simulink model "Practica1_InmanArturoArmasSalas"  (R2024a)
settings: Solver=ode23  StartTime=0.0  StopTime=10  RelTol=1e-3
values from neighbouring files (symbols this model uses):
  g = 9.81    [ParametrosPendulo.m]    (also in condiciones.m)
  l1 = 0.3    [ParametrosPendulo.m]    (also in condiciones.m)
  l2 = 0.25    [ParametrosPendulo.m]    (also in condiciones.m)
  m1 = 0.2    [ParametrosPendulo.m]    (also in condiciones.m)
  m2 = 0.1    [ParametrosPendulo.m]    (also in condiciones.m)
settings Model: Creator=Charles  LastModifiedBy=Elasticsole57
settings SolverCC: AlgebraicLoopSolver=TrustRegion
settings DataIOCC: ReturnWorkspaceOutputs=off
settings DebuggingCC: UnconnectedInputMsg=warning  UnconnectedOutputMsg=warning  UnconnectedLineMsg=warning  ArithmeticOperatorsInVariantConditions=warning
settings ModelReferenceCC: EnableRefExpFcnMdlSchedulingChecks=on
settings SFSimCC: SimUseLocalCustomCode=off  CustomCodeUndefinedFunction=UseInterfaceOnly
settings RTWCC: RTWUseLocalCustomCode=off  GPUComputeCapability=3.5

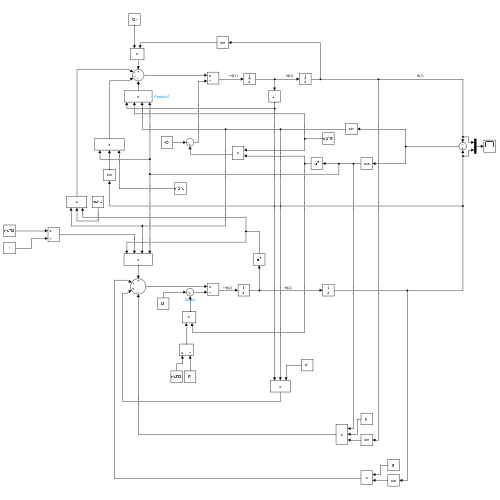
[thumbnail: Simulink's stored preview of the top-level diagram]
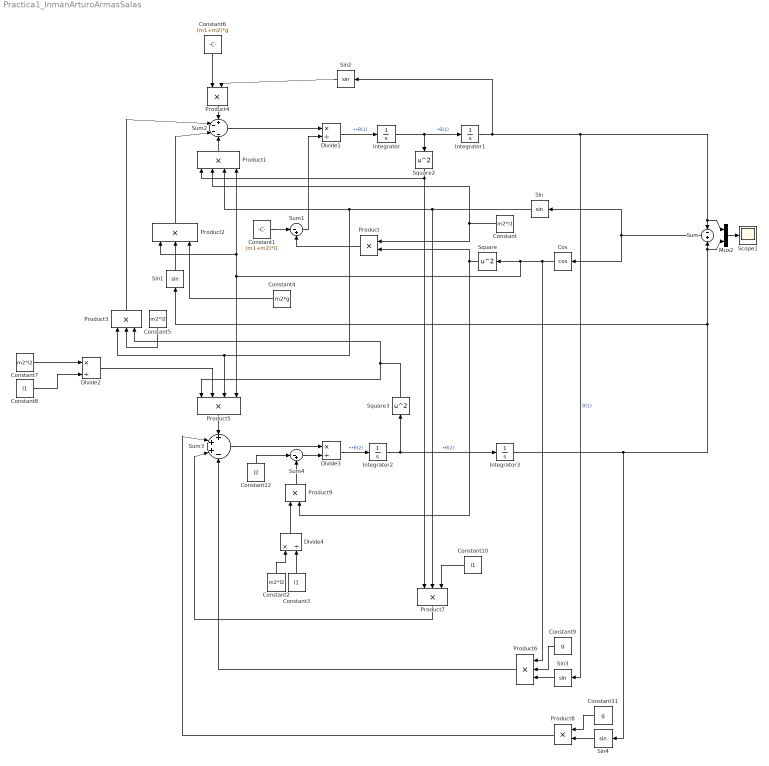
== system Practica1_InmanArturoArmasSalas ==
  Constant : Constant  Value=m2*l1
  Constant1 : Constant  Value=(m1+m2)*l1
  Constant10 : Constant  Value=l1
  Constant11 : Constant  Value=g
  Constant12 : Constant  Value=l2
  Constant2 : Constant  Value=m2*l2
  Constant3 : Constant  Value=l1
  Constant4 : Constant  Value=m2*g
  Constant5 : Constant  Value=m2*l2
  Constant6 : Constant  Value=(m1+m2)*g
  Constant7 : Constant  Value=m2*l2
  Constant8 : Constant  Value=l1
  Constant9 : Constant  Value=g
  Cos : Trigonometry  Operator=cos
  Divide{1..4} (4 alike) : Product  Inputs=*/
  Integrator : Integrator
  Integrator1 : Integrator
  Integrator2 : Integrator
  Integrator3 : Integrator  InitialCondition=0.610865
  Mux2 : Mux  Inputs=2
  Product{,4,8..9} (4 alike) : Product
  Product1 : Product  Inputs=4
  Product{2..3,6..7} (4 alike) : Product  Inputs=3
  Product5 : Product  Inputs=4
  Scope1 : Scope
  Sin{,1..4} (5 alike) : Trigonometry
  Square : Math  Operator=square  SignedPower=on  RndMeth=Zero
  Square2 : Math  Operator=square  SignedPower=on  RndMeth=Zero
  Square3 : Math  Operator=square  SignedPower=on  RndMeth=Zero
  Sum : Sum  Inputs=-+
  Sum1 : Sum  Inputs=|-+
  Sum2 : Sum  Inputs=+---
  Sum3 : Sum  Inputs=+++-
  Sum4 : Sum  Inputs=|-+
  wires:
  Integrator/1 -> Integrator1/1, Square2/1  "•θ(1)"
  Integrator1/1 -> Sin3/1, Mux2/1, Sum/1, Sin2/1  "θ(1)"
  Integrator2/1 -> Integrator3/1, Square3/1  "•θ(2)"
  Integrator3/1 -> Mux2/2, Sum/2, Sin1/1, Sin4/1
  Sum/1 -> Sin/1, Cos/1
  Cos/1 -> Product2/1, Product1/4, Product5/4, Square/1, Product6/1
  Sin/1 -> Product1/3, Product5/3, Product3/1, Product7/2
  Square/1 -> Product9/2, Product/2
  Constant/1 -> Product/1, Product1/2
  Constant1/1 -> Sum1/1
  Product/1 -> Sum1/2
  Sum1/1 -> Divide1/2
  Divide1/1 -> Integrator/1  "••θ(1)"
  Square2/1 -> Product7/1, Product1/1
  Product1/1 -> Sum2/4
  Sin1/1 -> Product2/2
  Constant4/1 -> Product2/3
  Product2/1 -> Sum2/3
  Constant5/1 -> Product3/2
  Square3/1 -> Product5/1, Product3/3
  Product3/1 -> Sum2/2
  Sin2/1 -> Product4/2
  Constant6/1 -> Product4/1
  Product4/1 -> Sum2/1
  Divide2/1 -> Product5/2
  Product5/1 -> Sum3/1
  Sin3/1 -> Product6/3
  Constant9/1 -> Product6/2
  Constant10/1 -> Product7/3
  Product7/1 -> Sum3/3
  Product6/1 -> Sum3/4
  Sin4/1 -> Product8/2
  Constant11/1 -> Product8/1
  Product8/1 -> Sum3/2
  Divide3/1 -> Integrator2/1  "••θ(2)"
  Constant2/1 -> Divide4/1
  Constant3/1 -> Divide4/2
  Product9/1 -> Sum4/2
  Constant12/1 -> Sum4/1
  Sum4/1 -> Divide3/2
  Mux2/1 -> Scope1/1
  Sum2/1 -> Divide1/1
  Sum3/1 -> Divide3/1
  Divide4/1 -> Product9/1
  Constant8/1 -> Divide2/2
  Constant7/1 -> Divide2/1
